simulink model "ReplayFlight_SensorMcu"  (Simulink 6.6)
settings: Solver=FixedStepDiscrete  StartTime=0.0  StopTime=time(end)  FixedStep=.01  RelTol=1e-3
InitFcn:
  | replayFlight
values from neighbouring files (symbols this model uses):
  apSampleTime = 0.01    [replayFlight.m]
  baroOffset = P(2)    [replayFlight.m]
  baroScale = P(1)    [replayFlight.m]
  baseHeight = 225    [replayFlight.m]
  baseTemp = 288.215    [replayFlight.m]
  cubeAccelGain = (2.522e-3)*9.815    (= 0.02475343)    [replayFlight.m]
  cubeGyroGain = .07326*pi/180    (= 0.00127862821001)    [replayFlight.m]
  GS_location = [0 36.9898376464844 -122.051963806152]    [replayFlight.m]
  lapseRate = -0.00198122    [replayFlight.m]
  magMeanTemp = [162.42 162.42 162.42]    [replayFlight.m]
  magOffset = 0    [replayFlight.m]
  magScale = 0.3418    [replayFlight.m]
  magTempK = [.0057 -.0423 .0426]    [replayFlight.m]
  pitotOffset = -1083.881038056753    (= -1083.88103806)    [replayFlight.m]
  pitotScale = 1.213292590242    (= 1.21329259024)    [replayFlight.m]
  powerOffset = P(2)    [replayFlight.m]
  powerScale = P(1)    [replayFlight.m]
  T = 0.01    [replayFlight.m]
  tempOffset = P(2)    [replayFlight.m]
  tempScale = P(1)    [replayFlight.m]
  Vb_0 = [ 25; 0;0]'    [replayFlight.m]
undefined symbols (not defined in the file or in its folder): baroMeanTemp, baroTempK, DiscIntNeverNeededParam, gaind, param_acc, param_mag, pitMeanTemp, pitTempK, polesd, q_quat, zerosd
libraries: aerolibconvert2 x10, simulink x8, SLUGS_Library x6, aerolibutil x4, dspmtrx3 x1, dsPICdrivers x1
(part 3 of 3)

== system ReplayFlight_SensorMcu/Sensor Data/Sensor Suite/Low Pass Filtering,Temperature Compensation and Calibration/Thermistor Unit Conversion ==
  Raw : Inport
  Bias : Constant  Value=bias  OutDataTypeMode=single
  Divide : Product  OutDataTypeMode=single  OutScaling=2^-10
  Gains : Constant  Value=gains  OutDataTypeMode=single
  Sum : Sum  Inputs=|++  OutDataTypeMode=single
  Comp : Outport
  wires:
  Bias/1 -> Sum/2
  Raw/1 -> Divide/2
  Gains/1 -> Divide/1
  Divide/1 -> Sum/1
  Sum/1 -> Comp/1

== system ReplayFlight_SensorMcu/Sensor Data/Sensor Suite/Low Pass Filtering,Temperature Compensation and Calibration/ValidateMags ==
  In1 : Inport
  Hold if Outlier : Subsystem  TreatAsAtomicUnit=on
  Monitor Norm : Subsystem
  Out1 : Outport
  wires:
  Hold if Outlier/1(Out1) -> Out1/1
  Monitor Norm/1(Enable) -> Hold if Outlier/Enable
  In1/1 -> Hold if Outlier/1(In1), Monitor Norm/1(Mags)

== system ReplayFlight_SensorMcu/Position and Attitude Filter/Attitude Complimentary Filter/Normalize Vector1/Norm/Subsystem3 ==
  x : Inport
  y : Inport  Port=2
  Embedded MATLAB Function : Stateflow chart
  x dot y : Outport
  wires:
  Embedded MATLAB Function/1(xDoty) -> x dot y/1
  x/1 -> Embedded MATLAB Function/1(x)
  y/1 -> Embedded MATLAB Function/2(y)

== system ReplayFlight_SensorMcu/Position and Attitude Filter/Attitude Complimentary Filter/Normalize Vector2/Norm/Subsystem3 ==
  x : Inport
  y : Inport  Port=2
  Embedded MATLAB Function : Stateflow chart
  x dot y : Outport
  wires:
  y/1 -> Embedded MATLAB Function/2(y)
  x/1 -> Embedded MATLAB Function/1(x)
  Embedded MATLAB Function/1(xDoty) -> x dot y/1

== system ReplayFlight_SensorMcu/Position and Attitude Filter/Geod2LTP1/ECEF2LTP (UEN)/From Body to Universal1/Rotation Matrix from Long//Lat ==
  note: Calculate Coefficients of DCM Row-Wise
  long lat : Inport
  11 : Fcn  Expr=cos(u[1])*cos(u[2])
  12 : Fcn  Expr=sin(u[1])*cos(u[2])
  13 : Fcn  Expr=sin(u[2])
  21 : Fcn  Expr=-sin(u[1])
  22 : Fcn  Expr=cos(u[1])
  23 : Fcn  Expr=0
  31 : Fcn  Expr=-sin(u[2])*cos(u[1])
  32 : Fcn  Expr=-sin(u[1])*sin(u[2])
  33 : Fcn  Expr=cos(u[2])
  Mux2 : Mux  Inputs=9
  DCM : Outport  InitialOutput=0
  wires:
  33/1 -> Mux2/9
  23/1 -> Mux2/8
  13/1 -> Mux2/7
  32/1 -> Mux2/6
  22/1 -> Mux2/5
  12/1 -> Mux2/4
  31/1 -> Mux2/3
  21/1 -> Mux2/2
  11/1 -> Mux2/1
  Mux2/1 -> DCM/1
  long lat/1 -> 11/1, 33/1, 23/1, 13/1, 32/1, 22/1, 12/1, 31/1, 21/1

== system ReplayFlight_SensorMcu/Sensor Data/Sensor Suite/Cube Signal Cond/3D Filter/Filter1 ==
  In1 : Inport
  Discrete Zero-Pole : DiscreteZeroPole  Zeros=zerosd  Poles=polesd  Gain=gaind  SampleTime=SampleTime
  Out1 : Outport
  wires:
  In1/1 -> Discrete Zero-Pole/1
  Discrete Zero-Pole/1 -> Out1/1

== system ReplayFlight_SensorMcu/Sensor Data/Sensor Suite/Cube Signal Cond/3D Filter/Filter2 ==
  In1 : Inport
  Discrete Zero-Pole : DiscreteZeroPole  Zeros=zerosd  Poles=polesd  Gain=gaind  SampleTime=SampleTime
  Out1 : Outport
  wires:
  Discrete Zero-Pole/1 -> Out1/1
  In1/1 -> Discrete Zero-Pole/1

== system ReplayFlight_SensorMcu/Sensor Data/Sensor Suite/Cube Signal Cond/3D Filter/Filter3 ==
  In1 : Inport
  Discrete Zero-Pole : DiscreteZeroPole  Zeros=zerosd  Poles=polesd  Gain=gaind  SampleTime=SampleTime
  Out1 : Outport
  wires:
  In1/1 -> Discrete Zero-Pole/1
  Discrete Zero-Pole/1 -> Out1/1

== system ReplayFlight_SensorMcu/Sensor Data/Sensor Suite/Cube Signal Cond/3D Filter1/Filter1 ==
  In1 : Inport
  Discrete Zero-Pole : DiscreteZeroPole  Zeros=zerosd  Poles=polesd  Gain=gaind  SampleTime=SampleTime
  Out1 : Outport
  wires:
  Discrete Zero-Pole/1 -> Out1/1
  In1/1 -> Discrete Zero-Pole/1

== system ReplayFlight_SensorMcu/Sensor Data/Sensor Suite/Cube Signal Cond/3D Filter1/Filter2 ==
  In1 : Inport
  Discrete Zero-Pole : DiscreteZeroPole  Zeros=zerosd  Poles=polesd  Gain=gaind  SampleTime=SampleTime
  Out1 : Outport
  wires:
  In1/1 -> Discrete Zero-Pole/1
  Discrete Zero-Pole/1 -> Out1/1

== system ReplayFlight_SensorMcu/Sensor Data/Sensor Suite/Cube Signal Cond/3D Filter1/Filter3 ==
  In1 : Inport
  Discrete Zero-Pole : DiscreteZeroPole  Zeros=zerosd  Poles=polesd  Gain=gaind  SampleTime=SampleTime
  Out1 : Outport
  wires:
  Discrete Zero-Pole/1 -> Out1/1
  In1/1 -> Discrete Zero-Pole/1

== system ReplayFlight_SensorMcu/Sensor Data/Sensor Suite/Low Pass Filtering,Temperature Compensation and Calibration/3D Filter/Filter1 ==
  In1 : Inport
  Discrete Zero-Pole : DiscreteZeroPole  Zeros=zerosd  Poles=polesd  Gain=gaind  SampleTime=SampleTime
  Out1 : Outport
  wires:
  In1/1 -> Discrete Zero-Pole/1
  Discrete Zero-Pole/1 -> Out1/1

== system ReplayFlight_SensorMcu/Sensor Data/Sensor Suite/Low Pass Filtering,Temperature Compensation and Calibration/3D Filter/Filter2 ==
  In1 : Inport
  Discrete Zero-Pole : DiscreteZeroPole  Zeros=zerosd  Poles=polesd  Gain=gaind  SampleTime=SampleTime
  Out1 : Outport
  wires:
  Discrete Zero-Pole/1 -> Out1/1
  In1/1 -> Discrete Zero-Pole/1

== system ReplayFlight_SensorMcu/Sensor Data/Sensor Suite/Low Pass Filtering,Temperature Compensation and Calibration/3D Filter/Filter3 ==
  In1 : Inport
  Discrete Zero-Pole : DiscreteZeroPole  Zeros=zerosd  Poles=polesd  Gain=gaind  SampleTime=SampleTime
  Out1 : Outport
  wires:
  In1/1 -> Discrete Zero-Pole/1
  Discrete Zero-Pole/1 -> Out1/1

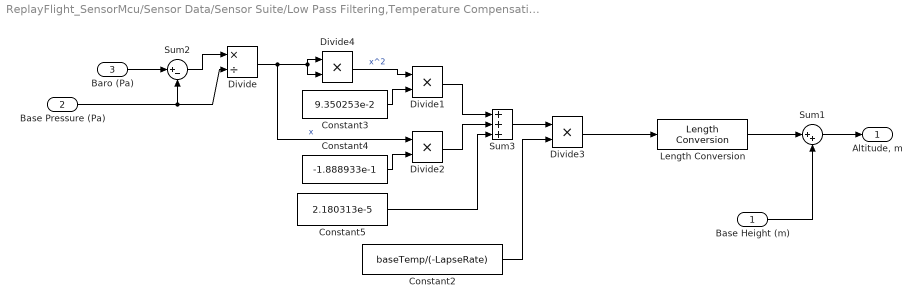
== system ReplayFlight_SensorMcu/Sensor Data/Sensor Suite/Low Pass Filtering,Temperature Compensation and Calibration/Baro Altimeter/Compute Barometric Height ==
  Base Height (m) : Inport
  Base Pressure (Pa) : Inport  Port=2
  Baro (Pa) : Inport  Port=3
  Constant2 : Constant  Value=baseTemp/(-LapseRate)  OutDataTypeMode=single
  Constant3 : Constant  Value=9.350253e-2  OutDataTypeMode=single
  Constant4 : Constant  Value=-1.888933e-1  OutDataTypeMode=single
  Constant5 : Constant  Value=2.180313e-5  OutDataTypeMode=single
  Divide : Product  Inputs=*/  OutDataTypeMode=single  OutScaling=2^-10
  Divide{1..4} (4 alike) : Product  OutDataTypeMode=single  OutScaling=2^-10
  Length Conversion : aerolibconvert2/Length Conversion  SystemSampleTime=-1  IU=ft  OU=m
  Sum1 : Sum  Inputs=|++  OutDataTypeMode=single
  Sum2 : Sum  Inputs=|+-  OutDataTypeMode=single
  Sum3 : Sum  Inputs=3  OutDataTypeMode=single
  "Altitude, m" : Outport
  wires:
  Baro (Pa)/1 -> Sum2/1
  Base Height (m)/1 -> Sum1/2
  Base Pressure (Pa)/1 -> Sum2/2, Divide/2
  Divide/1 -> Divide4/2, Divide4/1, Divide2/1  "x"
  Divide4/1 -> Divide1/1  "x^2"
  Constant3/1 -> Divide1/2
  Constant4/1 -> Divide2/2
  Divide1/1 -> Sum3/1
  Divide2/1 -> Sum3/2
  Constant5/1 -> Sum3/3
  Sum3/1 -> Divide3/1
  Constant2/1 -> Divide3/2
  Divide3/1 -> Length Conversion/1
  Sum1/1 -> "Altitude, m"/1
  Sum2/1 -> Divide/1
  Length Conversion/1 -> Sum1/1

== system ReplayFlight_SensorMcu/Sensor Data/Sensor Suite/Low Pass Filtering,Temperature Compensation and Calibration/Baro Altimeter/Enabled Subsystem ==
  In1 : Inport
  Enable : EnablePort
  Out1 : Outport  InitialOutput=baseHeight
  wires:
  In1/1 -> Out1/1

== system ReplayFlight_SensorMcu/Sensor Data/Sensor Suite/Low Pass Filtering,Temperature Compensation and Calibration/Baro Altimeter/Initial Baro Bias ==
  Baro (Pa) : Inport
  Enable : EnablePort
  Data Type Conversion : DataTypeConversion  OutDataTypeMode=double
  Data Type Conversion1 : DataTypeConversion  OutDataTypeMode=single
  Low Pass8 : Subsystem  mask(DiscretizedZeroPole){Zeros=[], Poles=[-3], Gain=3, AbsTol=auto, SampleTime=.01, method=tustin, Wc=1}
      mask prompts: Zeros "Zeros (enter in s-main:)"; Poles "Poles (enter in s-domain:)"; Gain "Gain (enter in s-domain:)"; AbsTol "Absolute tolerance:"; SampleTime "Sample time:"; Wc "Critical Frequency (Hz):"
      mask help: Continuous mask uses c2d to transform parameters onto the Discrete Zero-Pole block inside.
      mask init: same as ReplayFlight_SensorMcu/Low Pass1
      mask StyleString: edit,edit,edit,edit,edit,popup(zoh|foh|tustin|prewarp|matched),edit
      mask CallbackString: |||||hidecrit|
      mask Display:
      | droots(zeross,poless,gainss)
      | text( 0.5, 1.0, method, 'verticalAlignment','top')
  Mux : Mux  Inputs=2
  Scope : Scope
      settings: SaveName=ScopeData8
  "[80k - 120k]" : Saturate  UpperLimit=120000  LowerLimit=80000
  Baro (Gnd) : Outport
  wires:
  "[80k - 120k]"/1 -> Mux/1, Baro (Gnd)/1
  Mux/1 -> Scope/1
  Data Type Conversion1/1 -> "[80k - 120k]"/1, Mux/2
  Data Type Conversion/1 -> Low Pass8/1(In1)
  Low Pass8/1(Out1) -> Data Type Conversion1/1
  Baro (Pa)/1 -> Data Type Conversion/1

== system ReplayFlight_SensorMcu/Sensor Data/Sensor Suite/Low Pass Filtering,Temperature Compensation and Calibration/Baro Altimeter/Zero Out Height ==
  Base Height : Inport
  Computed Height : Inport  Port=2
  Enable : EnablePort
  Integer Delay : simulink/Discrete/Integer Delay  vinit=0  samptime=.01  NumDelays=1
  Sum : Sum  Inputs=|+-  OutDataTypeMode=single
  Height Offset : Outport
  wires:
  Base Height/1 -> Sum/1
  Integer Delay/1 -> Sum/2
  Sum/1 -> Height Offset/1
  Computed Height/1 -> Integer Delay/1

== system ReplayFlight_SensorMcu/Sensor Data/Sensor Suite/Low Pass Filtering,Temperature Compensation and Calibration/ValidateMags/Hold if Outlier ==
  In1 : Inport
  Enable : EnablePort
  Out1 : Outport  OutputWhenDisabled=reset  InitialOutput=[0 0 0]
  wires:
  In1/1 -> Out1/1

== system ReplayFlight_SensorMcu/Sensor Data/Sensor Suite/Low Pass Filtering,Temperature Compensation and Calibration/ValidateMags/Monitor Norm ==
  Mags : Inport
  0.7 < Norm < 1.5 : Subsystem
  Norm : Subsystem  AncestorBlock=SLUGS_Library/Navigation/Norm
  Enable : Outport
  wires:
  Mags/1 -> Norm/1(Vector)
  0.7 < Norm < 1.5/1(flag) -> Enable/1
  Norm/1(Norm) -> 0.7 < Norm < 1.5/1(norm)

== system ReplayFlight_SensorMcu/Sensor Data/Sensor Suite/Low Pass Filtering,Temperature Compensation and Calibration/Baro Altimeter/Initial Baro Bias/Low Pass8 ==
  In1 : Inport
  Discrete Zero-Pole : DiscreteZeroPole  Zeros=zerosd  Poles=polesd  Gain=gaind  SampleTime=SampleTime
  Out1 : Outport
  wires:
  Discrete Zero-Pole/1 -> Out1/1
  In1/1 -> Discrete Zero-Pole/1

== system ReplayFlight_SensorMcu/Sensor Data/Sensor Suite/Low Pass Filtering,Temperature Compensation and Calibration/ValidateMags/Monitor Norm/0.7 < Norm < 1.5 ==
  norm : Inport
  Compare To Constant : simulink/Logic and Bit Operations/Compare To Constant  SystemSampleTime=-1  relop=>  const=0.5  LogicOutDataTypeMode=uint8  ZeroCross=off
  Compare To Constant1 : simulink/Logic and Bit Operations/Compare To Constant  SystemSampleTime=-1  relop=<  const=1.6  LogicOutDataTypeMode=uint8  ZeroCross=off
  Logical Operator : Logic  AllPortsSameDT=off  OutDataTypeMode=Boolean
  flag : Outport
  wires:
  Logical Operator/1 -> flag/1
  norm/1 -> Compare To Constant1/1, Compare To Constant/1
  Compare To Constant/1 -> Logical Operator/1
  Compare To Constant1/1 -> Logical Operator/2

== system ReplayFlight_SensorMcu/Sensor Data/Sensor Suite/Low Pass Filtering,Temperature Compensation and Calibration/ValidateMags/Monitor Norm/Norm ==
  Vector : Inport
  Subsystem1 : Subsystem  AncestorBlock=SLUGS_Library/Subsystem1
  Subsystem3 : Subsystem  AncestorBlock=SLUGS_Library/Subsystem3
  Norm : Outport
  wires:
  Subsystem3/1(x dot y) -> Subsystem1/1(x)
  Vector/1 -> Subsystem3/2(y), Subsystem3/1(x)
  Subsystem1/1(sqrt(x)) -> Norm/1

== system ReplayFlight_SensorMcu/Sensor Data/Sensor Suite/Low Pass Filtering,Temperature Compensation and Calibration/ValidateMags/Monitor Norm/Norm/Subsystem1 ==
  x : Inport
  C Function Call : dsPICdrivers/OTHERS/C Function Call  Tag=dsPIC_dsPIC_CFunctionCall  fctName='mySqrt'  INPUT_SIZE=1  INPUT1=real32  INPUT2=--  INPUT3=--  OUTPUT_SIZE=1  OUTPUT1=real32  SampleTime=-1  InputType=[ 7 ]  OutputType=[ 7 ]  FctDeclaration=extern real32_T mySqrt(real32_T u1);  FctCall=%y1 = mySqrt(%u1);  OrderingInOutPopup=None
  negprotect : Stateflow chart
  sqrt(x) : Outport
  wires:
  C Function Call/1 -> sqrt(x)/1
  negprotect/1(zpVal) -> C Function Call/1
  x/1 -> negprotect/1(val)

== system ReplayFlight_SensorMcu/Sensor Data/Sensor Suite/Low Pass Filtering,Temperature Compensation and Calibration/ValidateMags/Monitor Norm/Norm/Subsystem3 ==
  x : Inport
  y : Inport  Port=2
  Embedded MATLAB Function : Stateflow chart
  x dot y : Outport
  wires:
  y/1 -> Embedded MATLAB Function/2(y)
  x/1 -> Embedded MATLAB Function/1(x)
  Embedded MATLAB Function/1(xDoty) -> x dot y/1

== matlab function Position and Attitude Filter/Attitude Complimentary Filter/Normalize Vector2/Norm/Subsystem3/Embedded MATLAB Function ==
  data: x input inherited; y input inherited; xDoty output inherited
function xDoty = myDot(x,y)
% This block supports an embeddable subset of the MATLAB language.
% See the help menu for details. 

xDoty = x(1)*y(1) + x(2)*y(2) + x(3)*y(3);

== matlab function Sensor Data/Sensor Suite/Cube Signal Cond/3D Filter/myMux Fun1 ==
  data: u1 input inherited; y output inherited; u2 input inherited; u3 input inherited
function y = myMux(u1, u2, u3)
% This block supports an embeddable subset of the MATLAB language.
% See the help menu for details. 

y = [u1(1); u2(1); u3(1)];

== matlab function Sensor Data/Sensor Suite/Cube Signal Cond/3D Filter1/myMux Fun1 ==
  data: u1 input inherited; y output inherited; u2 input inherited; u3 input inherited
function y = myMux(u1, u2, u3)
% This block supports an embeddable subset of the MATLAB language.
% See the help menu for details. 

y = [u1(1); u2(1); u3(1)];

== matlab function Sensor Data/Sensor Suite/Low Pass Filtering,Temperature Compensation and Calibration/3D Filter/myMux Fun1 ==
  data: u1 input inherited; y output inherited; u2 input inherited; u3 input inherited
function y = myMux(u1, u2, u3)
% This block supports an embeddable subset of the MATLAB language.
% See the help menu for details. 

y = [u1(1); u2(1); u3(1)];

== matlab function Position and Attitude Filter/Attitude Complimentary Filter/3D Filter/myMux Fun1 ==
  data: u1 input inherited; y output inherited; u2 input inherited; u3 input inherited
function y = myMux(u1, u2, u3)
% This block supports an embeddable subset of the MATLAB language.
% See the help menu for details. 

y = [u1(1); u2(1); u3(1)];

== matlab function Sensor Data/Sensor Suite/Low Pass Filtering,Temperature Compensation and Calibration/Baro Altimeter/Enables/Disables the Computation of initial Baro Bias ==
  data: tOut output inherited
function tOut = getTIni

persistent aveCount;
persistent tIni;

if isempty(aveCount)
    aveCount =1;
    tIni = 1;
end;

if aveCount < 2500
    aveCount = aveCount + 1;
end

if aveCount == 2500
    tIni =0;
    aveCount = aveCount + 1;
end

tOut = tIni;

%if aveCount > 500
%    tIni = 0;
%end

% if isempty(aveCount)
%     aveCount =1;
%     initBias = [0.0 0.0 0.0]';
% end;
%     
% if (aveCount<10)
%     initBias = initBias+ Raw;
%     bias = initBias/aveCount;
%     aveCount = aveCount +1;
% end;
% 
% if (aveCount == 10)
%     initBias = initBias/(aveCount-1);
%     aveCount = 100;
% end;
% 
% if (aveCount == 100)
%     bias = initBias;
% end;

== matlab function Position and Attitude Filter/Attitude Complimentary Filter/Embedded MATLAB Function ==
  data: u input inherited; y output inherited
function y = TwoPi(u)
% This block supports an embeddable subset of the MATLAB language.
% See the help menu for details. 

if ( u < 0 )
    y = u + 2*pi;
else
    y = u;
end

== matlab function Position and Attitude Filter/Attitude Complimentary Filter/Normalize Vector1/Norm/Subsystem3/Embedded MATLAB Function ==
  data: x input inherited; y input inherited; xDoty output inherited
function xDoty = myDot(x,y)
% This block supports an embeddable subset of the MATLAB language.
% See the help menu for details. 

xDoty = x(1)*y(1) + x(2)*y(2) + x(3)*y(3);

== matlab function Position and Attitude Filter/Attitude Complimentary Filter/q dot calc ==
  data: q input inherited size=4; om_hat input inherited; q_dot output single size=4
function q_dot = qXom(q,om_hat)
% This block supports an embeddable subset of the MATLAB language.
% See the help menu for details. 

	s = q(1,1);
    v = q(2:4,1);
    q_dot = single(zeros(4,1));
    q_dot(1,1) = -.5*v'*om_hat;
    q_dot(2:4,1) =  .5*[ s    -v(3) v(2); ...
                        v(3)  s    -v(1); ...
                       -v(2) v(1) s]*om_hat;

== matlab function Position and Attitude Filter/Attitude Complimentary Filter/myMux Fun1 ==
  data: u1 input inherited; y output inherited; u2 input inherited; u3 input inherited
function y = myMux3(u1, u2, u3)
% This block supports an embeddable subset of the MATLAB language.
% See the help menu for details. 

y = [u1(1); u2(1); u3(1)];

== matlab function Sensor Data/Sensor Suite/Low Pass Filtering,Temperature Compensation and Calibration/ValidateMags/Monitor Norm/Norm/Subsystem3/Embedded MATLAB Function ==
  data: x input inherited; y input inherited; xDoty output inherited
function xDoty = myDot(x,y)
% This block supports an embeddable subset of the MATLAB language.
% See the help menu for details. 

xDoty = x(1)*y(1) + x(2)*y(2) + x(3)*y(3);

== matlab function Sensor Data/Sensor Suite/Low Pass Filtering,Temperature Compensation and Calibration/ValidateMags/Monitor Norm/Norm/Subsystem1/negprotect ==
  data: val input inherited; zpVal output inherited
function zpVal = negProt(val)
% This block supports an embeddable subset of the MATLAB language.
% See the help menu for details. 

if val >= single(0.001)
    zpVal = val;
else
    zpVal = single(0.001);
end

== matlab function Position and Attitude Filter/Attitude Complimentary Filter/Quaternions to Direction Cosine Matrix/Create Transformation Matrix/myMux Fun1 ==
  data: u1 input inherited; y output inherited; u2 input inherited; u3 input inherited; u4 input inherited; u5 input inherited; u6 input inherited; u7 input inherited; u8 input inherited; u9 input inherited
function y = myMux3(u1, u2, u3, u4, u5, u6, u7, u8, u9)
% This block supports an embeddable subset of the MATLAB language.
% See the help menu for details. 

y = [u1(1); u2(1); u3(1); u4(1); u5(1); u6(1); u7(1); u8(1); u9(1)];

== matlab function Sensor Data/Sensor Suite/If no HIL then Read all the Sensors/myMux Fun4 ==
  data: u1 input inherited; y output inherited; u2 input inherited; u3 input inherited; u4 input inherited; u5 input inherited; u6 input inherited; u7 input inherited; u8 input inherited; u9 input inherited; u10 input inherited; u11 input inherited; u12 input inherited; u13 input inherited
function y = sensMux(u1, u2,u3,u4,u5,u6,u7,u8, u9, u10, u11, u12, u13)
% This block supports an embeddable subset of the MATLAB language.
% See the help menu for details. 

y = [u1(1); u2(1); u3(1); u4(1); u5(1); u6(1); u7(1); u8(1); u9(1); u10(1); u11(1); u12(1); u13(1)];

== matlab function Position and Attitude Filter/Velocity/Position Kalman Filter ==
  data: A_sens input inherited size=3; Vxyd_hat output inherited size=3; GPS_XYD input inherited size=3; RLT2B input inherited size=[3 3]; COS_D input inherited size=1; SOG input inherited size=1; NewGPS input inherited size=1; Pxyd_hat output inherited size=3; apSampleTime parameter inherited size=1; acc_bias output inherited size=3
function [Vxyd_hat, Pxyd_hat, acc_bias] = PosKF(A_sens, GPS_XYD, RLT2B, COS_D, SOG, ...
    NewGPS, apSampleTime)

% This implements a 9 state filter estimating inertial positions and velocities from 
% GPS, accelerometer.

% 5 measurments: GPS(XYD), Vnorth Veast

persistent PMinus;
persistent xHatMinus;
persistent xHatPlus;
persistent ZC3;
persistent A;
persistent C;
persistent RAssumed;
persistent QAssumed;
persistent MaxDeltaAcc;
persistent NGPS;

%persistent DT;
%persistent t;
%persistent I3;
%persistent Z3;
%persistent g;


if (isempty(ZC3))
    %t = single(0);
    %g = single();
    %millig = single(9.81/1000);
    %Z3 = single(zeros(3));
    %I3 = single(eye(3));
    %PhMinus = single( [100 0; ...
    %                    0 100]);

    ZC3 = single(zeros(3,1));
    %DT = apSampleTime; %prediction interval, must match pulse generator
    
    PMinus = single( [10e6*eye(3) zeros(3) zeros(3); ...
                       zeros(3) 10e6*eye(3)  zeros(3); ...
                       zeros(3)  zeros(3)  ((.0981)^2)*eye(3)]); 
    PPlus = PMinus;
    xHatMinus = single([-200 0 -500   -25 -4 0   0 0 0]');
    xHatPlus = xHatMinus;
    %     9 state transition matrix
%     influence of acc bias inserted later in A(4:6,7:9)
    tauAccel = 300; % shaping filter for accelerations
    A = single([eye(3) apSampleTime*eye(3) zeros(3); ...
                zeros(3)   eye(3)     zeros(3); ...
                zeros(3)  zeros(3) eye(3)*exp(-apSampleTime/tauAccel)]);

%     C = single([ I3 Z3 Z3;
%                  Z3 I3  Z3] );
%     no altitude rate measurement
    C = single([ eye(3) zeros(3) zeros(3);
                 0 0 0 1 0 0 0 0 0;
                 0 0 0 0 1 0 0 0 0] );
             
    QP = (.1^2)/apSampleTime;  %position change for one second
    QV = apSampleTime*(.123)^2;  %velocity variance from accel white noise
    QB = 0;  %(.000133)^2; %from Gabe's email, ren's spreadsheet
    QAssumed = single( [ QP*eye(3)  zeros(3)     zeros(3); ...
                          zeros(3)    QV*eye(3)  zeros(3); ...
                          zeros(3)     zeros(3)    QB*eye(3)] );
    
    MaxDeltaAcc = single(.0148/tauAccel); %sigma_b/tau
    
%     GPS observation noise
%     the altitude values will be replaced later
%     the altitude and altitude rate observation variance 
%     in the 9 state filter are replaced
%     by the covariances of the altitude filter at each update
    RP = .3^2;
    RV = .1^2;
%     RAssumed = single( [ RP*I3  Z3; ...
%                         Z3  RV*I3] );
    RAssumed = single( [ RP 0 0  0  0; ...
                         0 RP 0  0  0;
                         0 0 RP  0  0;
                         0 0 0   RV 0 ;
                         0 0 0   0  RV ] );
                    
    NGPS = 0;
end

% wait for first GPS update
if( SOG <= 2)
    Vxyd_hat = xHatPlus(4:6);
    Pxyd_hat = xHatPlus(1:3) + apSampleTime*Vxyd_hat;
    acc_bias = xHatPlus(7:9);
%     t = t + apSampleTime;
%     if ( t > .9)
%         t
%     end
    
    return
end

if( NewGPS && SOG > 2)
%     if ( t > 74.5)
%         t
%     end
    
    Vn = cos(COS_D*pi/180)*SOG;
    Ve = sin(COS_D*pi/180)*SOG;
    z = single([GPS_XYD(1:3); Vn; Ve]);
    zHat = C*xHatMinus;
    % innovation
    innov = z - zHat;
    
%     process sequentially
    PPlus = PMinus; % dummy to avoid error messabe
    TotalDeltaxHat = single(zeros(9,1));
    for ii = 1:5
        Ci = single(C(ii,1:end));
        PCiT = PMinus*transpose(Ci);
        Ki = single(PCiT/( Ci*PCiT + RAssumed(ii,ii) ));
        PPlus = (single(eye(9)) - Ki*Ci)*PMinus;
        DeltaxHat = Ki*innov(ii);
        TotalDeltaxHat = TotalDeltaxHat + DeltaxHat;
        PMinus = PPlus;
    end
%     clip changes in bias to 1 mg per update
    for ii = 7:9
        TotalDeltaxHat(ii) = max(-MaxDeltaAcc, min(TotalDeltaxHat(ii), MaxDeltaAcc));
    end
    xHatPlus = xHatMinus + TotalDeltaxHat;
%     if NGPS = 0, set velocity to
%     measured velocity to avoid big jump due to position iniialization
    if (NGPS == 0 )
        xHatPlus(4:6) = [Vn;Ve;0];
    end
    NGPS = NGPS + 1;
else
%     no new GPS
    PPlus = PMinus;
    xHatPlus = xHatMinus;
end

% propogate to next time step
RB2LT = transpose(RLT2B);
A(4:6,7:9) = apSampleTime*RB2LT;
PMinus = A*PPlus*transpose(A) + QAssumed;
%ForceDT = apSampleTime*(RB2LT*A_sens + [0; 0; 9.81]);
ForceDT = ZC3;
xHatMinus = A*xHatPlus + [ ZC3; ...
                        ForceDT; ...
                          ZC3];
% if ( t > 59.1)
%     t
%    AB = apSampleTime*RB2LT*xHatPlus(7:9)
%    ForceDT
%    xHatMinus
% end

Pxyd_hat = xHatPlus(1:3);
Vxyd_hat = xHatPlus(4:6);
acc_bias = xHatPlus(7:9);

%t = t + apSampleTime;

== matlab function Sensor Data/Sensor Suite/Low Pass Filtering,Temperature Compensation and Calibration/Ellipse Correction/myMux Fun3 ==
  data: u1 input inherited; y output inherited; u2 input inherited; u3 input inherited
function y = myMux(u1, u2, u3)
% This block supports an embeddable subset of the MATLAB language.
% See the help menu for details. 

y = [u1(1); u2(1); u3(1)];

== matlab function Sensor Data/Sensor Suite/Cube Signal Cond/Ellipse Correction/myMux Fun3 ==
  data: u1 input inherited; y output inherited; u2 input inherited; u3 input inherited
function y = myMux(u1, u2, u3)
% This block supports an embeddable subset of the MATLAB language.
% See the help menu for details. 

y = [u1(1); u2(1); u3(1)];
